simulink model "SimpleTransmissionn"  (R2022b)
settings: Solver=VariableStepAuto  StartTime=0.0  StopTime=1000  RelTol=1e-3
libraries: commsequence2 x2, commdigbbndpm3 x2, dspsrcs4 x2, commfilt2 x2, commchan3 x1, simulink x1, commsink2 x1, commsync2 x1, dspsigops x1
(part 2 of 2)

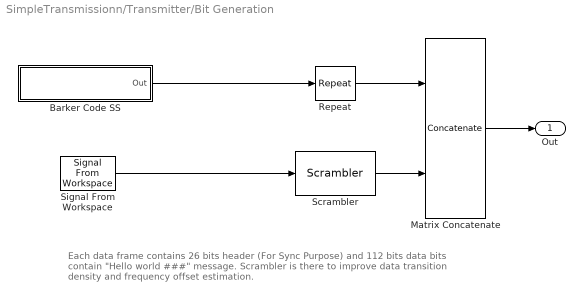
== system SimpleTransmissionn/Transmitter/Bit Generation ==
  note: Each data frame contains 26 bits header (For Sync Purpose) and 112 bits data bits
      | contain "Hello world ###" message. Scrambler is there to improve data
      | transition density and frequency offset estimation.
  Barker Code SS : Subsystem
      mask Display: disp('Unipolar\nBarker Code')
  Matrix Concatenate : Concatenate  Mode=Multidimensional array
  Repeat : dspsigops/Repeat  N=2  InputProcessing=Columns as channels (frame based)  RateOptions=Enforce single-rate processing  ic=0  mode=Unused parameter value
  Scrambler : commsequence2/Scrambler  M=2  poly=[1 1 1 0 1]  iniStaSource=Dialog Parameter  ini_sta=[1 0 0 0]  resetViaPort=off
  Signal From Workspace : dspsrcs4/Signal From Workspace  X="[1\t0\t0\t1\t0\t0\t0\t1\t1\t0\t0\t1\t0\t1\t1\t1\t0\t1\t1\t0\t0\t1\t1\t0\t1\t1\t0\t0\t1\t1\t0\t1\t1\t1\t1\t0\t1\t0\t0\t0\t0\t0\t1\t1\t1\t0\t1\t1\t1\t1\t1\t0\t1\t1\t1\t1\t1\t1\t1\t0\t0\t1\t0\t1\t1\t0\t1\t1\t0\t0\t1\t1\t0\t0\t1\t0\t0\t0\t1\t0\t0\t0\t0\t0\t0\t1\t1\t0\t0\t0\t0\t0\t1\t1\t0\t0\t0\t0\t0\t1\t1\t0\t0\t0\t0\t0\t0\t0\t1\t0\t1\t0\t1\t0\t0\t1\t0\t0\t0\t1\t1\t0\t0\t1\t0\t1\t1\t1\t0\t1\t1\t0\t0\t1 ...(+33198 chars)].'"  Ts=1.0116e-05  nsamps=2240  OutputAfterFinalValue=Cyclic repetition  ignoreOrWarnInputAndFrameLengths=on  OutputFrames=off
  Out : Outport  VectorParamsAs1DForOutWhenUnconnected=off
  wires:
  Barker Code SS/1(Out) -> Repeat/1
  Matrix Concatenate/1 -> Out/1
  Repeat/1 -> Matrix Concatenate/1
  Scrambler/1 -> Matrix Concatenate/2
  Signal From Workspace/1 -> Scrambler/1

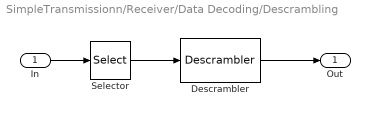
== system SimpleTransmissionn/Receiver/Data Decoding/Descrambling ==
  In : Inport
  Descrambler : commsequence2/Descrambler  M=2  poly=[1 1 1 0 1]  iniStaSource=Dialog Parameter  ini_sta=[1 0 0 0]  resetViaPort=off
  Selector : Selector  IndexOptions=Index vector (dialog)  Indices=[27:2266]  OutputSizes=1
  Out : Outport  VectorParamsAs1DForOutWhenUnconnected=off
  wires:
  In/1 -> Selector/1
  Selector/1 -> Descrambler/1
  Descrambler/1 -> Out/1

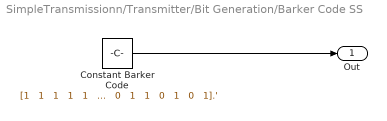
== system SimpleTransmissionn/Transmitter/Bit Generation/Barker Code SS ==
  Constant Barker Code : Constant  Value="[1   1   1   1   1   0   0   1   1   0   1   0   1].'"  VectorParams1D=off  OutDataTypeStr=double
  Out : Outport  VectorParamsAs1DForOutWhenUnconnected=off
  wires:
  Constant Barker Code/1 -> Out/1
